simulink model "DC_grid_V2"  (R2018a)
settings: Solver=VariableStepAuto  StartTime=0.0  StopTime=10  RelTol=1e-3
values from neighbouring files (symbols this model uses):
  inputsFromWS = Simulink.Parameter(inputArray)    [DC_grid.m]    (also in QlearningEMS_Average.m; init_for_DC_grid.m)
  Q = repmat(zeros(size(states,1),1,'single'),[1,3,3])    [QlearningEMS.m]    (also in QlearningEMS_Average.m = repmat(zeros(size(Q_states,1),1,'single'),[1,3]))
undefined symbols (not defined in the file or in its folder): Batt, BatteryCback, BatteryLoadFcn, Continuous, FC, FuelCellLoadFcn, gcbh, MC, sps_rtmsupport, spsBatteryModel
libraries: simulink x7, powerlib x6, spsFuelCellModel x1
settings Model: SimulationMode=accelerator  Creator=David Pasdeloup  LastModifiedBy=David Pasdeloup
settings DataIOCC: FinalStateName=myOperPoint  LoadInitialState=on  SaveFinalState=on  SaveCompleteFinalSimState=on

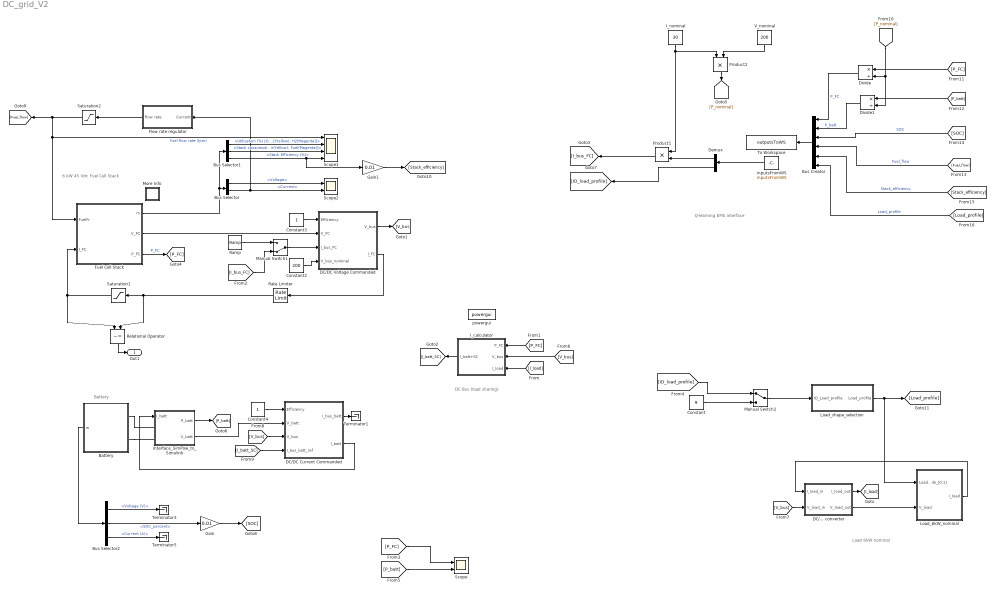
== system DC_grid_V2 ==
  note: 6 kW 45 Vdc Fuel Cell Stack
  note: Battery
  note: DC Bus (load sharing)
  note: Load 6kW nominal
  note: Q-learning EMS interface
  Battery : Subsystem  DialogController=POWERSYS.PowerSysDialog  LoadFcn=sps_rtmsupport('LoadFcn',gcbh); BatteryLoadFcn(gcb)  InitFcn=BatteryCback(gcb,1)  StartFcn=sps_rtmsupport('StartFcn',gcbh);  StopFcn=sps_rtmsupport('StopFcn',gcbh);  mask(Battery){BatType=Lithium-Ion, ShowTempParam=off, ThermalPreset=no, ShowAgeParam=off, NomV=MC.nominal_voltage, NomQ=MC.rated_capacity, SOC=MC.initial_SOC, Batt_Tr=MC.battery_response_time, PresetModel=off, MaxQ=1.5, MinV=75, FullV=116.3987, Dis_rate=64, R=0.66667, Normal_OP=1.3565, expZone=[108.0386    0.07369565], current=100, Units=Time, Tci=20, NomT=25, T2=0, MaxQ2=2.208, FullV2=3.45, Normal_OP2=2.8, expZone2=[3.22        0.23], Rca=0.6, ti=1000, Dp=0, Neq0=0, Tsim=1e6, Ta1=25, Qeol=5.4*0.9, Reol=0.013333*1.2, Char_age=[2.3478, 3], Dis_age=[2.3478, 10], N1=1500, N2=10500, N3=1000, N4=1400, Ta2=45, N5=950}
      mask prompts: BatType "Type:"; ShowTempParam "Simulate temperature effects"; ThermalPreset "Use a preset battery:"; ShowAgeParam "Simulate aging effects"; NomV "Nominal voltage (V)"; NomQ "Rated capacity (Ah)"; SOC "Initial state-of-charge (%)"; Batt_Tr "Battery response time (s)"; PresetModel "Determined from the nominal parameters of the battery"; MaxQ "Maximum capacity (Ah)"; MinV "Cut-off Voltage (V)"; FullV "Fully charged voltage (V)"; Dis_rate "Nominal discharge current (A)"; R "Internal resistance (Ohms)"; Normal_OP "Capacity (Ah) at nominal voltage"; expZone "Exponential zone [Voltage (V), Capacity (Ah)]"; current "Discharge current [i1, i2, i3,...] (A)"; Tci "Initial cell temperature (deg. C)"; NomT "Nominal ambient temperature T1 (deg. C)"; T2 "Second ambient temperature T2 (deg. C)"; MaxQ2 "Maximum capacity (Ah)"; FullV2 "Initial discharge voltage (V)"; Normal_OP2 "Voltage at 90% maximum capacity (V)"; expZone2 "Exponential zone [Voltage (V), Capacity (Ah)]"; Rca "Thermal resistance, cell-to-ambient (deg. C/W)"; ti "Thermal time constant, cell-to-ambient (s)"; Dp "Heat loss difference [charge vs. discharge] (W)"; Neq0 "Initial battery age (Equivalent full cycles)"; Tsim "Aging model sampling time (s)"; Ta1 "Ambient temperature Ta1 (deg. C)"; Qeol "Capacity at EOL (End Of Life) (Ah)"; Reol "Internal resistance at EOL (Ohms)"; Char_age "Charge current (nominal, maximum) [Ic (A), Icmax (A)]"; Dis_age "Discharge current (nominal, maximum) [Id (A), Idmax (A)]"; N1 "Cycle life at 100 % DOD, Ic and Id (Cycles)"; N2 "Cycle life at 25 % DOD, Ic and Id (Cycles)"; N3 "Cycle life at 100 % DOD, Ic and Idmax (Cycles)"; N4 "Cycle life at 100 % DOD, Icmax and Id (Cycles)"; Ta2 "Ambient temperature Ta2 (deg. C)"; N5 "Cycle life at 100 % DOD, Ic and Id (Cycles)"
      mask help: Implements a generic battery model for most popular battery types. Temperature and aging (due to cycling) effects can be specified for Lithium-Ion battery type.
      mask init:
      | block = gcb;
      | BatteryCback(block,3)
      | [Batt BT, WantBlockChoice, Ts] = BatteryParam(NomV,NomQ,MaxQ,MinV,FullV,Dis_rate,R,Normal_OP,expZone,block,0);
      | powericon('SetInternalModels','set',block,WantBlockChoice);
      | BatteryCback(block,1);
      | 
      | % Lines added by David Pasdeloup 27 June 2018
      | %disp('The battery model have been initialized now'); %flag to (un)comment
      settings: CopyFcn=sps_rtmsupport('CopyFcn',gcbh);  DeleteFcn=sps_rtmsupport('DeleteFcn',gcbh);  UndoDeleteFcn=sps_rtmsupport('UndoDeleteFcn',gcbh);  ModelCloseFcn=sps_rtmsupport('ModelCloseFcn',gcbh);  PreSaveFcn=sps_rtmsupport('PreSaveFcn',gcbh);  PostSaveFcn=sps_rtmsupport('PostSaveFcn',gcbh);  NameChangeFcn=sps_rtmsupport('NameChangeFcn',gcbh);  PreCopyFcn=sps_rtmsupport('PreCopyFcn',gcbh);  OpenFcn=sps_rtmsupport('OpenFcn',gcbh, [1,2,3,4,9,18]);  CloseFcn=sps_rtmsupport('CloseFcn',gcbh);  PreDeleteFcn=sps_rtmsupport('PreDeleteFcn',gcbh);
      mask Help: helpview(psbhelp)
      mask TypeOptions BatType: Lead-Acid | Lithium-Ion | Nickel-Cadmium | Nickel-Metal-Hydride
      mask Callback BatType: BatteryCback(gcb,1)
      mask Callback ShowTempParam: BatteryCback(gcb,1)
      mask TypeOptions ThermalPreset: no | 3.3V  2.3Ah  (LiFePO4) | 3.6V  2050mAh   (LiCoO2) | 3.6V  2.0Ah | 3.6V  3.6Ah  (LiNiO2) | 3.6V  4.5Ah | 3.6V  48Ah  (LiNiO2) | 3.7V  4.4Ah | 7.4V  5.4Ah  (LiCoO2) | 11.1V  6600mAh  (LiCoO2) | 12.8V  40Ah  (LiFeMgPO4)
      mask Callback ThermalPreset: BatteryCback(gcb,4)
      mask Callback ShowAgeParam: BatteryCback(gcb,1)
      mask Callback PresetModel: BatteryCback(gcb,1)
      mask TypeOptions Units: Ampere-hour | Time
      mask Callback ti: sps_rtmsupport('parametereditingmodes',gcbh, [1,2,3,4,9,18]);
      mask DialogControl ParameterTabVar0 Prompt: Parameters
      mask DialogControl Tempcontainer Prompt: Temperature
      mask DialogControl Agecontainer Prompt: Aging
      mask DialogControl ParameterTabVar01 Prompt: Discharge
      mask DialogControl Container9 Prompt: Display characteristics
      mask DialogControl PlotButton Prompt: Plot
      mask DialogControl PlotButton Callback: BatteryCback(gcb,0)
      mask DialogControl Temperature Prompt: Temperature
      mask DialogControl Container7 Prompt: Discharge parameters at T2
      mask DialogControl Container8 Prompt: Thermal response and Heat loss
      mask DialogControl Aging Prompt: Aging
      mask DialogControl Container16 Prompt: Aging characteristics at ambient temperature Ta1
      mask DialogControl Container13 Prompt: Aging characteristics at ambient temperature Ta2
      mask Display:
      | patch([BT.X1 BT.X1m],[BT.Y1 BT.Y1m],BT.color1);
      | patch(BT.X3,BT.Y3,BT.color2);
      | plot([BT.X1 BT.X1m BT.X2 BT.X2m BT.X3 BT.X4],[BT.Y1 BT.Y1m BT.Y2 BT.Y2m BT.Y3 BT.Y4]);
      | plot(-100,-60,60,50,[BT.X(1) BT.X(1)],[BT.bas BT.haut],[BT.X(2) BT.X(2)],[BT.haut BT.bas],BT.dim_Xsin,4*sin(BT.dim_sin)+BT.haut,BT.dim_Xsin,-4*sin(BT.dim_sin)+BT.haut,BT.dim_Xsin,-4*sin(BT.dim_sin)+BT.bas,BT.dim_Xtop,sin(BT.dim_top)+BT.haut+4,BT.dim_Xtop,-sin(BT.dim_top)+BT.haut+4,BT.dim_Xtop,-sin(BT.dim_top)+BT.haut,[BT.TopX(2),BT.TopX(2)],[BT.haut,BT.haut+4],[BT.TopX(1),BT.TopX(1)],[BT.haut+4,BT.haut]);plot(BT.dim_Xsin,-5*sin(BT.dim_sin)+20);
      | port_label('lconn',1,'+');
      | port_label('lconn',2,'_');
      | color('blue');
      | port_label('output',1,'m');
      | 
      | if Batt.sel_T
      |     port_label('input',1,'Ta');
      | end
  Bus Creator : BusCreator  Inputs=6
  Bus Selector : BusSelector  OutputSignals=Voltage,Current
  Bus Selector1 : BusSelector  OutputSignals=Utilization (%) [O2(Yellow); H2(Magenta)],Stack consumption (lpm) [Air(Yellow); Fuel(Magenta)],Stack Efficiency (%)
  Bus Selector2 : BusSelector  OutputSignals=Voltage (V),SOC_percent,Current (A)
  Constant : Constant  Value=9
  Constant2 : Constant  Value=200
  Constant3 : Constant
  Constant4 : Constant
  DC/... converter : Subsystem
  DC/DC Current Commanded : Subsystem
  DC/DC Voltage Commanded : Subsystem
  Demux : Demux  Outputs=2
  Divide : Product  Inputs=*/
  Divide1 : Product  Inputs=*/
  Flow rate regulator : Subsystem  mask{Nc=65, Uf_H2=99.56, T=65, Pf=1.5, x=99.95}
      mask prompts: Nc "Number of cells"; Uf_H2 "Nominal Hydrogen utilization (%)"; T "Operating temperature (Celsius)"; Pf "Fuel pressure (bar)"; x "H2 composition (%)"
  Fuel Cell Stack : Subsystem  DialogController=POWERSYS.PowerSysDialog  LoadFcn=sps_rtmsupport('LoadFcn',gcbh);FuelCellLoadFcn(gcb)  StartFcn=sps_rtmsupport('StartFcn',gcbh);  StopFcn=sps_rtmsupport('StopFcn',gcbh);  mask(Fuel Cell Stack){PresetModel=PEMFC - 6 kW - 45 Vdc, FcType=Proton Exchange Membrane (PEM), Detailed=Detailed, Eoc=[65,63], NomVI=[133.3,45], EndVI=[225,37], Nc=65, n=55, TOp=65, AirFr=300, SuppPress=[1.5,1], Comp=[99.95,21,1], SignX=off, SignY=off, FlowRateH2=on, FlowRateAir=off, SystemTemp=off, SystemPH2=off, SystemPAir=off, FCDyn=on, FC_tau=10, Peak_O2=80, V_Under=10}
      mask prompts: PresetModel "Preset model:"; FcType "Fuel Cell type:"; Detailed "Model detail Level:"; Eoc "Voltage at 0A and 1A [V_0(V), V_1(V)]"; NomVI "Nominal operating point [Inom(A), Vnom(V)]"; EndVI "Maximum operating point [Iend(A), Vend(V)]"; Nc "Number of cells"; n "Nominal stack efficiency (%)"; TOp "Operating temperature (Celsius)"; AirFr "Nominal Air flow rate (lpm)"; SuppPress "Nominal supply pressure [Fuel (bar), Air (bar)]"; Comp "Nominal composition (%) [H2 O2 H2O(Air)]"; SignX "Fuel  composition [x_H2(%)]"; SignY "Oxidant composition [y_O2(%)]"; FlowRateH2 "Fuel flow rate [FuelFr(lpm)]"; FlowRateAir "Air flow rate [AirFr(lpm)]"; SystemTemp "System Temperature [T(Kelvin)]"; SystemPH2 "Fuel supply pressure [Pfuel(bar)]"; SystemPAir "Air supply pressure [PAir(bar)]"; FCDyn "Specify Fuel Cell Dynamics?"; FC_tau "Fuel Cell response time (sec)"; Peak_O2 "Peak O2 utilization (%)"; V_Under "Voltage undershoot (V) @ peak O2 utilization"
      mask help:
      | Implements a generic hydrogen fuel cell model which allows the simulation for the following types of cells:
      | - Proton Exchange Membrane Fuel Cell (PEMFC)
      | - Solid Oxide Fuel Cell (SOFC)
      | - Alkaline Fuel Cell (AFC)
      mask init:
      | block = gcb;
      | %% DO NOT CHANGE THIS ORDER
      | FuelCellCback(block,'Inputs')
      | [FC, WantBlockChoice, Ts] = FuelCellInit(block,Eoc,NomVI,EndVI,Nc,n,TOp,AirFr,SuppPress,Comp,FlowRateH2,FlowRateAir);
      | powericon('SetInternalModels','set',block,WantBlockChoice);
      | 
      | % Added by David 27/06/2018. Uncomment this line to track when the 
      | % model is compilled:
      | %disp('FC has been initilaized');
      settings: CopyFcn=sps_rtmsupport('CopyFcn',gcbh);  DeleteFcn=sps_rtmsupport('DeleteFcn',gcbh);  UndoDeleteFcn=sps_rtmsupport('UndoDeleteFcn',gcbh);  ModelCloseFcn=sps_rtmsupport('ModelCloseFcn',gcbh);  PreSaveFcn=sps_rtmsupport('PreSaveFcn',gcbh);  PostSaveFcn=sps_rtmsupport('PostSaveFcn',gcbh);  NameChangeFcn=sps_rtmsupport('NameChangeFcn',gcbh);  PreCopyFcn=sps_rtmsupport('PreCopyFcn',gcbh);  OpenFcn=sps_rtmsupport('OpenFcn',gcbh, [1 2 3 13 14 15 16 17 18 19 20]);  CloseFcn=sps_rtmsupport('CloseFcn',gcbh);  PreDeleteFcn=sps_rtmsupport('PreDeleteFcn',gcbh);
      mask Help: helpview(psbhelp)
      mask TypeOptions PresetModel: No (User-Defined) | PEMFC - 1.26 kW - 24 Vdc | PEMFC - 6 kW - 45 Vdc | PEMFC - 50 kW - 625 Vdc | AFC - 2.4 kW - 48 Vdc | SOFC - 3 kW - 100 Vdc | SOFC - 25 kW - 630 Vdc
      mask Callback PresetModel: FuelCellCback(gcb,'Preset')
      mask TypeOptions Detailed: Simplified | Detailed
      mask Callback Detailed: FuelCellCback(gcb,'Visibilities')
      mask Callback FlowRateAir: FuelCellCback(gcb,'Visibilities')
      mask Callback FCDyn: FuelCellCback(gcb,'Visibilities')
      mask DialogControl ParameterTabVar0 Prompt: Parameters
      mask DialogControl plot_graph Prompt: Plot V_I characteristic
      mask DialogControl plot_graph Callback: FuelCellCback(gcb,'PlotGraph');
      mask DialogControl ViewParam Prompt: View Cell parameters
      mask DialogControl ViewParam Callback: FuelCellCback(gcb,'ViewParam');
      mask DialogControl ParameterTabVar01 Prompt: Signal variation
      mask DialogControl ParameterTabVar012 Prompt: Fuel Cell Dynamics
      mask Display: image(imread('power_fuelcell.png'));
  Gain : Gain  Gain=0.01
  Gain1 : Gain  Gain=0.01
  I_calculator : Subsystem
  I_nominal : Constant  Value=30
  Interface_SimPow_to_Simulink : Subsystem
  Load_6kW_nominal : Subsystem
  Load_shape_selection : Subsystem
  Manual Switch1 : ManualSwitch  CurrentSetting=0
  Manual Switch2 : ManualSwitch
  More Info : Subsystem
      settings: OpenFcn=showdemo(bdroot(gcb))
      mask Display: disp('?')
  Product1 : Product
  Product2 : Product
  Ramp : simulink/Sources/Ramp  slope=5  start=10  InitialOutput=0
  Rate Limiter : RateLimiter  RisingSlewLimit=8  FallingSlewLimit=-8  SampleTimeMode=inherited
  Relational Operator : RelationalOperator  Operator=~=  OutDataTypeStr=boolean  RndMeth=Simplest
  Saturation1 : Saturate  UpperLimit=225  LowerLimit=0
  Saturation2 : Saturate  UpperLimit=85  LowerLimit=0
  Scope : Scope  NumInputPorts=2
  Scope1 : Scope  NumInputPorts=4
  Scope2 : Scope  NumInputPorts=2
  Terminator1 : Terminator
  Terminator3 : Terminator
  Terminator5 : Terminator
  To Workspace : ToWorkspace  VariableName=outputsToWS  SaveFormat=Timeseries  SampleTime=-1
  V_nominal : Constant  Value=200
  inputsFromWS : Constant  Value=inputsFromWS
  powergui : powerlib/powergui  SimulationMode=Continuous  SampleTime=1e-6  frequency=60  Iterations=50  frequencyindice=0  Pbase=100e6  ErrMax=1e-4  UnitsV=kV  UnitsW=MW  buscounter=0  FunctionMessages=off  echomessages=off  EnableUseOfTLC=off  CurrentSourceSwitches=off  DisableSnubberDevices=off  DisableRonSwitches=off  DisableVfSwitches=off  DisplayEquations=off  SolverType=Tustin/Backward Euler (TBE)  Interpol=off  ExternalGateDelay=off  methode=off  Ts=100  x0status=blocks  SPID=on  SwTol=0  HookPort=off  RestoreLinks=warning  ResistiveCurrentMeasurement=off  Frange=[0:2:500]  Ylog=off  Xlog=on  ShowGrid=off  save=off  variable=ZData  structure=0  ZoomFFT=on  StartTime=0.0  cycles=1  DisplayStyle=1  fundamental=60  FreqAxis=off  MaxFrequency=1000  frequencyindicesteady=1  RmsSteady=1  display=off
  Out1 : Outport
  wires:
  Battery/1(m) -> Bus Selector2/1
  Constant2/1 -> DC/DC Voltage Commanded/4(V_bus_nominal)
  [I_bus_FC] -> Manual Switch1/2
  Constant/1 -> Manual Switch2/2
  Manual Switch1/1 -> DC/DC Voltage Commanded/3(I_bus_FC)
  [ID_load_profile] -> Manual Switch2/1
  Interface_SimPow_to_Simulink/1(P_batt) -> [P_batt]
  Fuel Cell Stack/1(m) -> Bus Selector/1, Bus Selector1/1
  Load_6kW_nominal/1(I_load) -> DC/... converter/1(I_load_in)
  Saturation1/1 -> Relational Operator/1, Fuel Cell Stack/2(I_FC)
  [I_load] -> I_calculator/3(I_load)
  Relational Operator/1 -> Out1/1
  DC/... converter/1(I_load_out) -> [I_load]
  Rate Limiter/1 -> Relational Operator/2, Saturation1/1
  Constant3/1 -> DC/DC Voltage Commanded/1(Efficiency)
  Bus Selector1/1 -> Scope1/2  "<Utilization (%) [O2(Yellow); H2(Magenta)]>"
  Ramp/1 -> Manual Switch1/1
  DC/DC Voltage Commanded/2(I_FC) -> Rate Limiter/1
  Bus Selector1/2 -> Scope1/3  "<Stack consumption (lpm) [Air(Yellow); Fuel(Magenta)]>"
  DC/... converter/2(V_load_out) -> Load_6kW_nominal/2(V_load)
  Fuel Cell Stack/3(P_FC) -> [P_FC]  "P_FC"
  Saturation2/1 -> [Fuel_flow], Fuel Cell Stack/1(FuelFr), Scope1/1  "Fuel flow rate (lpm)"
  Bus Selector1/3 -> Gain1/1, Scope1/4  "<Stack Efficiency (%)>"
  Bus Selector/2 -> Flow rate regulator/1(Current), Scope2/2  "<Current>"
  Bus Selector/1 -> Scope2/1  "<Voltage>"
  Flow rate regulator/1(flow rate) -> Saturation2/1
  Bus Selector2/3 -> Terminator5/1  "<Current (A)>"
  Bus Selector2/2 -> Gain/1  "<SOC_percent>"
  Bus Selector2/1 -> Terminator3/1  "<Voltage (V)>"
  [P_FC] -> Scope/1
  [P_batt] -> Scope/2
  Constant4/1 -> DC/DC Current Commanded/1(Efficiency)
  Interface_SimPow_to_Simulink/2(V_batt) -> DC/DC Current Commanded/2(V_batt)
  DC/DC Current Commanded/2(I_batt) -> Interface_SimPow_to_Simulink/1(I_batt)
  DC/DC Current Commanded/1(I_bus_batt) -> Terminator1/1
  [P_FC] -> I_calculator/1(P_FC)
  DC/DC Voltage Commanded/1(V_bus) -> [V_bus]
  [V_bus] -> I_calculator/2(V_bus)
  Fuel Cell Stack/2(V_FC) -> DC/DC Voltage Commanded/2(V_FC)
  [V_bus] -> DC/... converter/2(V_load_in)
  [V_bus] -> DC/DC Current Commanded/3(V_bus)
  I_calculator/1(I_batt+SC) -> [I_batt_SC]
  [I_batt_SC] -> DC/DC Current Commanded/4(I_bus_batt_ref)
  Demux/1 -> Product1/2
  Demux/2 -> [ID_load_profile]
  Bus Creator/1 -> To Workspace/1
  [P_batt] -> Divide1/1
  Divide1/1 -> Bus Creator/2  "P_batt"
  inputsFromWS/1 -> Demux/1
  Product1/1 -> [I_bus_FC]
  Divide/1 -> Bus Creator/1  "P_FC"
  Product2/1 -> [P_nominal]
  [P_nominal] -> Divide1/2, Divide/2
  V_nominal/1 -> Product2/2
  [P_FC] -> Divide/1
  I_nominal/1 -> Product1/1, Product2/1
  [SOC] -> Bus Creator/3  "SOC"
  Gain/1 -> [SOC]
  Gain1/1 -> [Stack_efficiency]
  [Fuel_flow] -> Bus Creator/4  "Fuel_flow"
  [Stack_efficiency] -> Bus Creator/5  "Stack_efficiency"
  Manual Switch2/1 -> Load_shape_selection/1(ID_Load_profile)
  Load_shape_selection/1(Load_profile) -> [Load_profile], Load_6kW_nominal/1(Load_profile_[0;1])
  [Load_profile] -> Bus Creator/6  "Load_profile"
  connections:
  Battery/LConn2 -- Interface_SimPow_to_Simulink/LConn2
  Battery/LConn1 -- Interface_SimPow_to_Simulink/LConn1

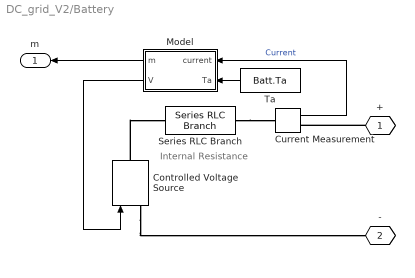
== system DC_grid_V2/Battery ==
  note: Internal Resistance
  Controlled Voltage Source : powerlib/Electrical Sources/Controlled Voltage Source  Initialize=on  Source_Type=AC  Amplitude=0  Phase=0  Frequency=0  Measurements=None
  Current Measurement : powerlib/Measurements/Current Measurement  PhasorSimulation=off  OutputType=Complex  PSBequivalent=0
  Model : Subsystem  AncestorBlock=spsBatteryModel/Continuous
  Series RLC Branch : powerlib/Elements/Series RLC Branch  LConnTagsString=__new0  RConnTagsString=__new0  BranchType=R  Resistance=Batt.R  Inductance=1e-3  SetiL0=off  InitialCurrent=0  Capacitance=1e-6  Setx0=off  InitialVoltage=0  Measurements=None
  Ta : Constant  Value=Batt.Ta
  + : PMIOPort  Tag=PMCPort  Side=Left
  - : PMIOPort  Tag=PMCPort  Port=2  Side=Left
  m : Outport
  wires:
  Ta/1 -> Model/2(Ta)
  Current Measurement/1 -> Model/1(current)  "Current"
  Model/1(m) -> m/1
  Model/2(V) -> Controlled Voltage Source/1
  connections:
  Series RLC Branch/RConn1 -- Current Measurement/LConn1
  Controlled Voltage Source/RConn1 -- Series RLC Branch/LConn1
  Controlled Voltage Source/LConn1 -- -/RConn1
  +/RConn1 -- Current Measurement/RConn1

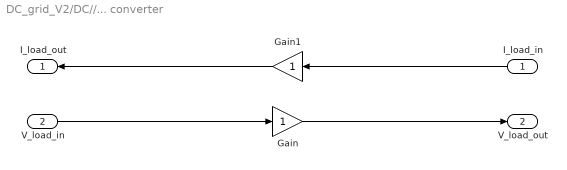
== system DC_grid_V2/DC//... converter ==
  I_load_in : Inport
  V_load_in : Inport  Port=2
  Gain : Gain
  Gain1 : Gain
  I_load_out : Outport
  V_load_out : Outport  Port=2
  wires:
  I_load_in/1 -> Gain1/1
  Gain/1 -> V_load_out/1
  Gain1/1 -> I_load_out/1
  V_load_in/1 -> Gain/1

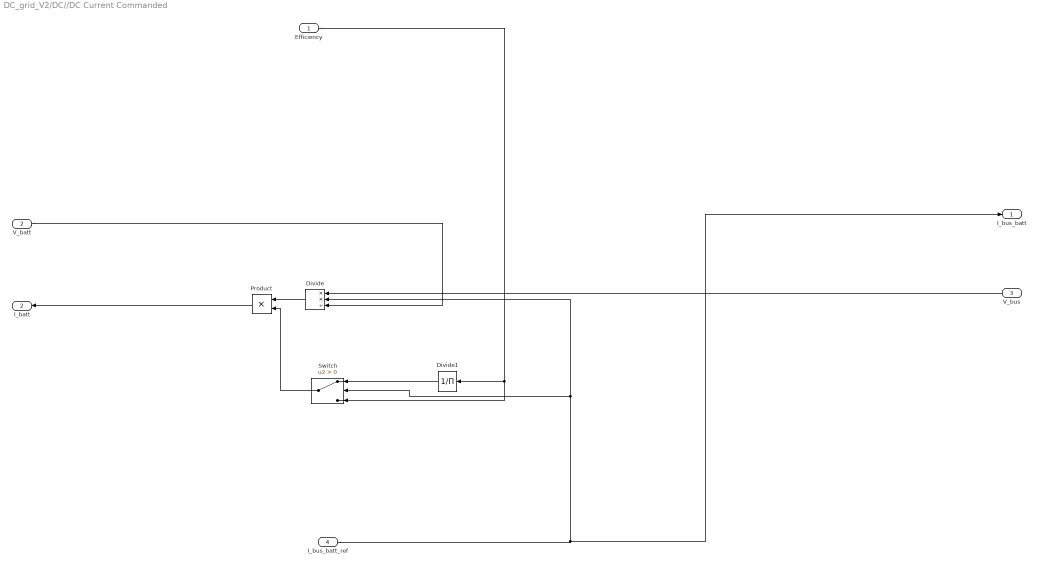
== system DC_grid_V2/DC//DC Current Commanded ==
  Efficiency : Inport
  V_batt : Inport  Port=2
  V_bus : Inport  Port=3
  I_bus_batt_ref : Inport  Port=4
  Divide : Product  Inputs=**/
  Divide1 : Product  Inputs=/
  Product : Product
  Switch : Switch  Criteria=u2 > Threshold
  I_bus_batt : Outport
  I_batt : Outport  Port=2
  wires:
  I_bus_batt_ref/1 -> Divide/2, Switch/2, I_bus_batt/1
  V_bus/1 -> Divide/1
  V_batt/1 -> Divide/3
  Efficiency/1 -> Divide1/1, Switch/3
  Divide1/1 -> Switch/1
  Divide/1 -> Product/1
  Switch/1 -> Product/2
  Product/1 -> I_batt/1

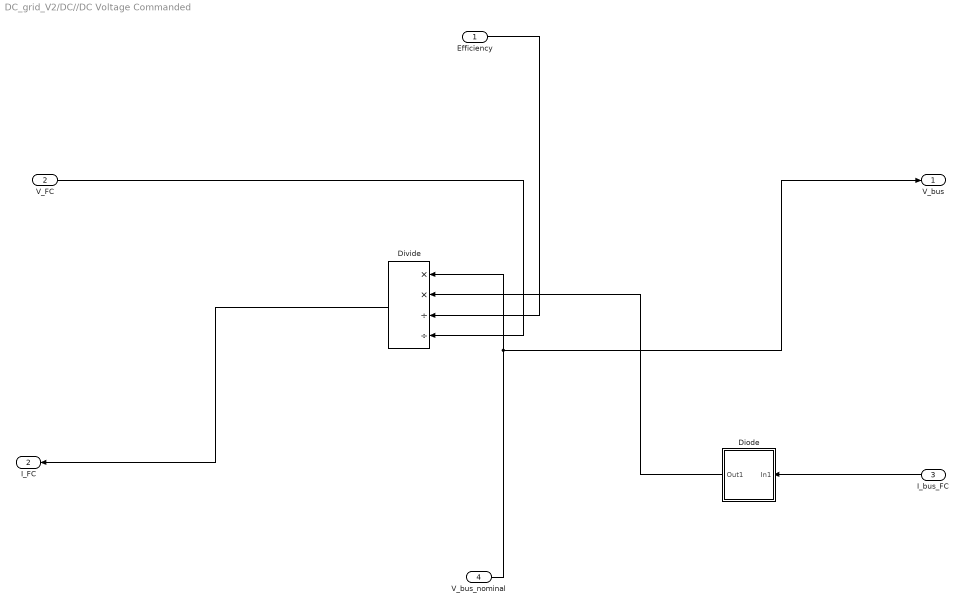
== system DC_grid_V2/DC//DC Voltage Commanded ==
  Efficiency : Inport
  V_FC : Inport  Port=2
  I_bus_FC : Inport  Port=3
  V_bus_nominal : Inport  Port=4
  Diode : Subsystem
  Divide : Product  Inputs=**//
  V_bus : Outport
  I_FC : Outport  Port=2
  wires:
  V_bus_nominal/1 -> V_bus/1, Divide/1
  V_FC/1 -> Divide/4
  Divide/1 -> I_FC/1
  Efficiency/1 -> Divide/3
  I_bus_FC/1 -> Diode/1(In1)
  Diode/1(Out1) -> Divide/2

== system DC_grid_V2/Flow rate regulator ==
  Current : Inport
  Fcn1 : Fcn  Expr=60000*8.3145*(273+T)*Nc*u(1)/(2*96485*(Pf*101325)*Uf_H2/100*x/100)
  Saturation : Saturate  UpperLimit=inf  LowerLimit=1
  flow rate : Outport
  wires:
  Fcn1/1 -> Saturation/1
  Current/1 -> Fcn1/1
  Saturation/1 -> flow rate/1

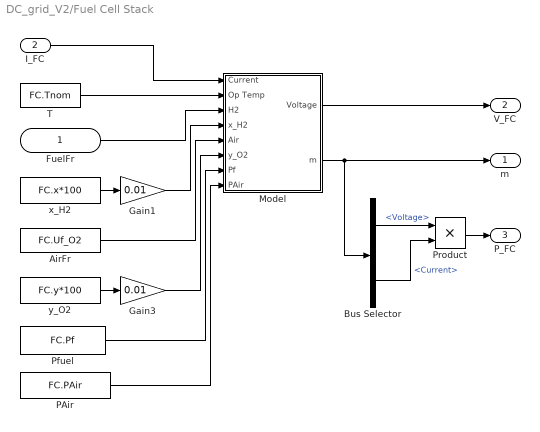
== system DC_grid_V2/Fuel Cell Stack ==
  FuelFr : Inport
  I_FC : Inport  Port=2
  AirFr : Constant  Value=FC.Uf_O2
  Bus Selector : BusSelector  OutputSignals=Voltage,Current
  Gain1 : Gain  Gain=0.01
  Gain3 : Gain  Gain=0.01
  Model : Subsystem  BlockChoice=Continuous/Detailed
      settings: AttributesFormatString=%<BlockChoice>  TemplateBlock=spsFuelCellModel/Fuel Cell model  MemberBlocks=Continuous/Detailed,Continuous/Simplified,Discrete/Detailed,Discrete/Simplified
  PAir : Constant  Value=FC.PAir
  Pfuel : Constant  Value=FC.Pf
  Product : Product
  T : Constant  Value=FC.Tnom
  x_H2 : Constant  Value=FC.x*100
  y_O2 : Constant  Value=FC.y*100
  m : Outport
  V_FC : Outport  Port=2
  P_FC : Outport  Port=3
  wires:
  PAir/1 -> Model/8(PAir)
  Pfuel/1 -> Model/7(Pf)
  T/1 -> Model/2(Op Temp)
  Model/1(Voltage) -> V_FC/1
  Model/2(m) -> Bus Selector/1, m/1
  FuelFr/1 -> Model/3(H2)
  x_H2/1 -> Gain1/1
  AirFr/1 -> Model/5(Air)
  y_O2/1 -> Gain3/1
  Gain1/1 -> Model/4(x_H2)
  Gain3/1 -> Model/6(y_O2)
  I_FC/1 -> Model/1(Current)
  Bus Selector/1 -> Product/1  "<Voltage>"
  Bus Selector/2 -> Product/2  "<Current>"
  Product/1 -> P_FC/1

== system DC_grid_V2/I_calculator ==
  P_FC : Inport
  V_bus : Inport  Port=2
  I_load : Inport  Port=3
  Add : Sum  Inputs=-+
  Divide : Product  Inputs=*/
  I_batt+SC : Outport
  wires:
  I_load/1 -> Add/2
  Divide/1 -> Add/1
  P_FC/1 -> Divide/1
  V_bus/1 -> Divide/2
  Add/1 -> I_batt+SC/1

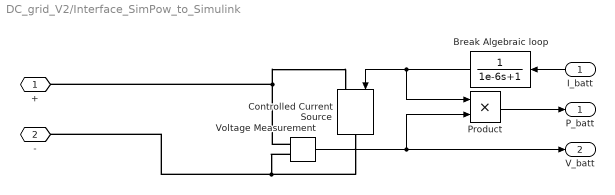
== system DC_grid_V2/Interface_SimPow_to_Simulink ==
  I_batt : Inport
  Break Algebraic loop : TransferFcn  Denominator=[1e-6 1]
  Controlled Current Source : powerlib/Electrical Sources/Controlled Current Source  Initialize=off  Source_Type=DC  Amplitude=0  Phase=0  Frequency=0  Measurements=None
  Product : Product
  Voltage Measurement : powerlib/Measurements/Voltage Measurement  PhasorSimulation=off  OutputType=Complex  PSBequivalent=0
  + : PMIOPort  Side=Left
  - : PMIOPort  Port=2  Side=Left
  P_batt : Outport
  V_batt : Outport  Port=2
  wires:
  Product/1 -> P_batt/1
  I_batt/1 -> Break Algebraic loop/1
  Voltage Measurement/1 -> V_batt/1, Product/2
  Break Algebraic loop/1 -> Product/1, Controlled Current Source/1
  connections:
  Voltage Measurement/LConn2 -- Controlled Current Source/RConn1 -- -/RConn1
  Voltage Measurement/LConn1 -- Controlled Current Source/LConn1 -- +/RConn1

== system DC_grid_V2/Load_6kW_nominal ==
  Load_profile_[0;1] : Inport
  V_load : Inport  Port=2
  I=P/U : Product  Inputs=*/
  Nominal_load_power : Constant  Value=6000
  Product : Product
  I_load : Outport
  wires:
  Load_profile_[0;1]/1 -> Product/2
  Product/1 -> I=P/U/1
  Nominal_load_power/1 -> Product/1
  V_load/1 -> I=P/U/2
  I=P/U/1 -> I_load/1

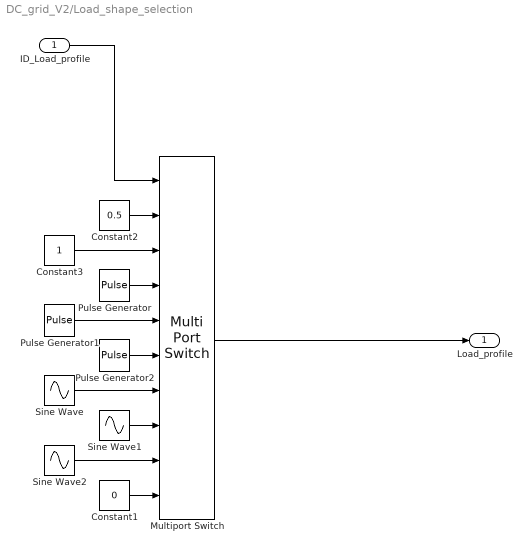
== system DC_grid_V2/Load_shape_selection ==
  ID_Load_profile : Inport
  Constant1 : Constant  Value=0
  Constant2 : Constant  Value=0.5
  Constant3 : Constant
  Multiport Switch : MultiPortSwitch  DataPortOrder=Specify indices  DataPortIndices={1,2,3,4,5,6,7,8,9}
  Pulse Generator : DiscretePulseGenerator  PulseType=Time based  Period=1  PulseWidth=50  PhaseDelay=10
  Pulse Generator1 : DiscretePulseGenerator  PulseType=Time based  Period=5  PulseWidth=50  PhaseDelay=10
  Pulse Generator2 : DiscretePulseGenerator  PulseType=Time based  Period=60  PulseWidth=50  PhaseDelay=10
  Sine Wave : Sin  Amplitude=0.5  Bias=0.5  Frequency=2*pi  Phase=-pi/2  SampleTime=0
  Sine Wave1 : Sin  Amplitude=0.5  Bias=0.5  Frequency=2*pi/5  Phase=-pi/2  SampleTime=0
  Sine Wave2 : Sin  Amplitude=0.5  Bias=0.5  Frequency=2*pi/60  Phase=-pi/2  SampleTime=0
  Load_profile : Outport
  wires:
  Constant1/1 -> Multiport Switch/10
  Sine Wave2/1 -> Multiport Switch/9
  Pulse Generator2/1 -> Multiport Switch/6
  Sine Wave/1 -> Multiport Switch/7
  Constant2/1 -> Multiport Switch/2
  Constant3/1 -> Multiport Switch/3
  Pulse Generator1/1 -> Multiport Switch/5
  Pulse Generator/1 -> Multiport Switch/4
  Sine Wave1/1 -> Multiport Switch/8
  Multiport Switch/1 -> Load_profile/1
  ID_Load_profile/1 -> Multiport Switch/1

== system DC_grid_V2/More Info ==

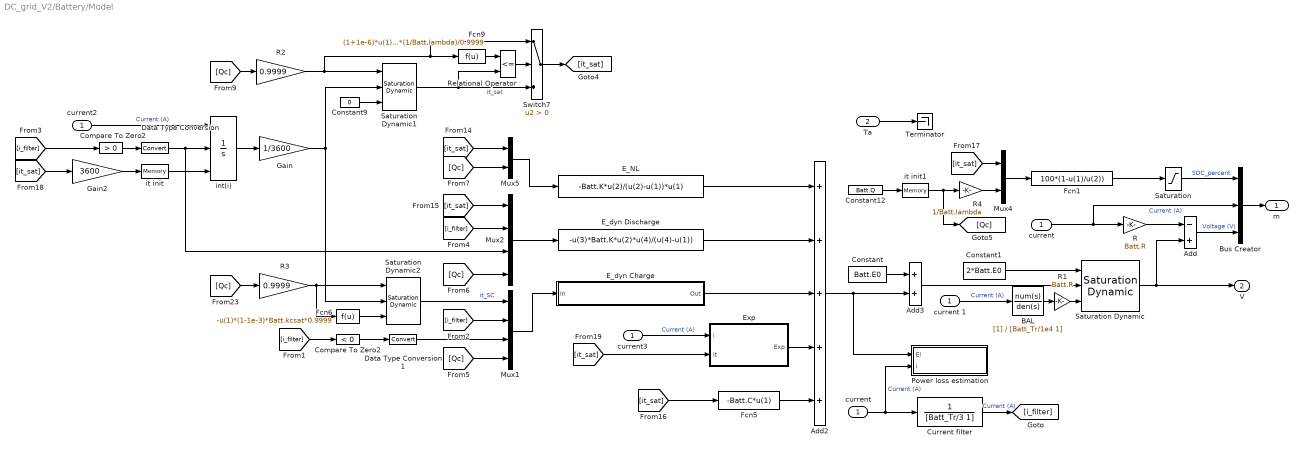
== system DC_grid_V2/Battery/Model ==
  current : Inport
  Ta : Inport  Port=2
  Add : Sum  Inputs=-+
  Add2 : Sum  Inputs=+++++
  Add3 : Sum
  BAL : TransferFcn  Denominator=[Batt_Tr/1e4 1]
  Bus Creator : BusCreator  Inputs=3
  Compare To Zero : simulink/Logic and Bit Operations/Compare To Zero  relop=>  OutDataTypeStr=uint8
  Compare To Zero2 : simulink/Logic and Bit Operations/Compare To Zero  relop=<  OutDataTypeStr=uint8
  Constant : Constant  Value=Batt.E0
  Constant1 : Constant  Value=2*Batt.E0
  Constant12 : Constant  Value=Batt.Q
  Constant9 : Constant  Value=0
  Current filter : TransferFcn  Denominator=[Batt_Tr/3 1]
  Data Type Conversion1 : DataTypeConversion
  Data Type Conversion2 : DataTypeConversion
  E_NL : Fcn  Expr=-Batt.K*u(2)/(u(2)-u(1))*u(1)
  E_dyn Charge : Subsystem
  E_dyn Discharge : Fcn  Expr=-u(3)*Batt.K*u(2)*u(4)/(u(4)-u(1))
  Exp : Subsystem
  Fcn1 : Fcn  Expr=100*(1-u(1)/u(2))
  Fcn5 : Fcn  Expr=-Batt.C*u(1)
  Fcn6 : Fcn  Expr=-u(1)*(1-1e-3)*Batt.kcsat*0.9999
  Fcn9 : Fcn  Expr=(1+1e-6)*u(1)*(1/Batt.lambda)/0.9999
  Gain : Gain  Gain=1/3600
  Gain2 : Gain  Gain=3600
  Mux1 : Mux
  Mux2 : Mux
  Mux4 : Mux  Inputs=2
  Mux5 : Mux  Inputs=2
  Power loss estimation : Subsystem
  R : Gain  Gain=Batt.R
  R1 : Gain  Gain=Batt.R
  R2 : Gain  Gain=0.9999
  R3 : Gain  Gain=0.9999
  R4 : Gain  Gain=1/Batt.lambda
  Relational Operator : RelationalOperator  Operator=<=  RndMeth=Simplest
  Saturation : Saturate  UpperLimit=100  LowerLimit=0
  Saturation Dynamic : simulink/Discontinuities/Saturation Dynamic  OutMin=[]  OutMax=[]  OutDataTypeStr=Inherit: Same as second input  OutDataType=sfix(16)  OutScaling=2^-10  DoSatur=off
  Saturation Dynamic1 : simulink/Discontinuities/Saturation Dynamic  OutMin=[]  OutMax=[]  OutDataTypeStr=Inherit: Same as second input  OutDataType=sfix(16)  OutScaling=2^-10  DoSatur=off
  Saturation Dynamic2 : simulink/Discontinuities/Saturation Dynamic  OutMin=[]  OutMax=[]  OutDataTypeStr=Inherit: Same as second input  OutDataType=sfix(16)  OutScaling=2^-10  DoSatur=off
  Switch7 : Switch  Criteria=u2 > Threshold
  Terminator : Terminator
  "current " : InportShadow
  current 1 : InportShadow
  current2 : InportShadow
  current3 : InportShadow
  int(i) : Integrator  ExternalReset=rising  InitialConditionSource=external  InitialCondition=(1-SOC/100)*Q*3600  LimitOutput=on  UpperSaturationLimit=Batt.Qmax*3600
  it init : Memory  InitialCondition=(1-SOC/100)*Batt.Q*(1/Batt.lambda)*3600
  it init1 : Memory  InitialCondition=Batt.Q
  m : Outport
  V : Outport  Port=2
  wires:
  BAL/1 -> R1/1
  current 1/1 -> BAL/1  "Current (A)"
  Constant12/1 -> it init1/1
  Constant1/1 -> Saturation Dynamic/1
  Ta/1 -> Terminator/1
  current/1 -> R/1, Bus Creator/2  "Current (A)"
  int(i)/1 -> Gain/1
  Fcn1/1 -> Saturation/1
  Add/1 -> Bus Creator/3  "Voltage (V)"
  R/1 -> Add/1
  Bus Creator/1 -> m/1
  Mux2/1 -> E_dyn Discharge/1
  Constant/1 -> Add3/1
  Mux1/1 -> E_dyn Charge/1(In)
  it init/1 -> int(i)/3
  Compare To Zero/1 -> Data Type Conversion2/1
  Compare To Zero2/1 -> Data Type Conversion1/1
  Data Type Conversion2/1 -> Mux2/3, int(i)/2
  Gain2/1 -> it init/1
  Exp/1(Exp) -> Add2/4
  Data Type Conversion1/1 -> Mux1/3
  Saturation Dynamic2/1 -> Mux1/1  "it_SC"
  Add3/1 -> Saturation Dynamic/2
  E_dyn Discharge/1 -> Add2/2
  E_NL/1 -> Add2/1
  E_dyn Charge/1(Out) -> Add2/3
  Fcn5/1 -> Add2/5
  Mux4/1 -> Fcn1/1
  Mux5/1 -> E_NL/1
  Fcn6/1 -> Saturation Dynamic2/3
  current2/1 -> int(i)/1  "Current (A)"
  current3/1 -> Exp/1(i)  "Current (A)"
  "current "/1 -> Current filter/1, Power loss estimation/2(i)  "Current (A)"
  [i_filter] -> Compare To Zero2/1
  [i_filter] -> Mux1/2
  [i_filter] -> Compare To Zero/1
  [i_filter] -> Mux2/2
  [Qc] -> Mux1/4
  [Qc] -> Mux2/4
  it init1/1 -> R4/1, [Qc]
  [Qc] -> R2/1
  [it_sat] -> Mux5/1
  [it_sat] -> Mux2/1
  [it_sat] -> Fcn5/1
  [it_sat] -> Mux4/1
  [it_sat] -> Gain2/1
  [it_sat] -> Exp/2(it)
  [Qc] -> R3/1
  R3/1 -> Fcn6/1, Saturation Dynamic2/1
  Add2/1 -> Add3/2, Power loss estimation/1(El)
  R4/1 -> Mux4/2
  Saturation/1 -> Bus Creator/1  "SOC_percent"
  Saturation Dynamic/1 -> Add/2, V/1
  [Qc] -> Mux5/2
  Gain/1 -> Saturation Dynamic1/2, Saturation Dynamic2/2
  Constant9/1 -> Saturation Dynamic1/3
  Current filter/1 -> [i_filter]  "Current (A)"
  R1/1 -> Saturation Dynamic/3
  Saturation Dynamic1/1 -> Relational Operator/2, Switch7/3  "it_sat"
  R2/1 -> Switch7/1, Fcn9/1, Saturation Dynamic1/1
  Switch7/1 -> [it_sat]
  Fcn9/1 -> Relational Operator/1
  Relational Operator/1 -> Switch7/2

== system DC_grid_V2/DC//DC Voltage Commanded/Diode ==
  In1 : Inport
  Constant : Constant  Value=0
  MinMax : MinMax  Function=max  Inputs=2
  Out1 : Outport
  wires:
  Constant/1 -> MinMax/2
  In1/1 -> MinMax/1
  MinMax/1 -> Out1/1

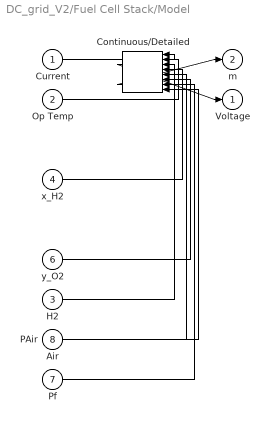
== system DC_grid_V2/Fuel Cell Stack/Model ==
  Current : Inport
  Op Temp : Inport  Port=2
  H2 : Inport  Port=3
  x_H2 : Inport  Port=4
  Air : Inport  Port=5
  y_O2 : Inport  Port=6
  Pf : Inport  Port=7
  PAir : Inport  Port=8
  Continuous/Detailed : spsFuelCellModel/Continuous//Detailed
  Voltage : Outport
  m : Outport  Port=2
  wires:
  Current/1 -> Continuous/Detailed/1
  Op Temp/1 -> Continuous/Detailed/2
  H2/1 -> Continuous/Detailed/3
  x_H2/1 -> Continuous/Detailed/4
  Air/1 -> Continuous/Detailed/5
  y_O2/1 -> Continuous/Detailed/6
  Pf/1 -> Continuous/Detailed/7
  PAir/1 -> Continuous/Detailed/8
  Continuous/Detailed/1 -> Voltage/1
  Continuous/Detailed/2 -> m/1

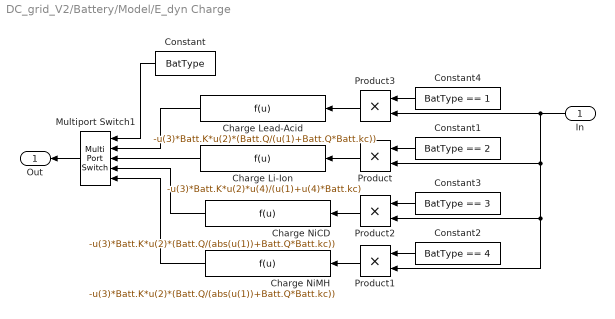
== system DC_grid_V2/Battery/Model/E_dyn Charge ==
  In : Inport
  Charge Lead-Acid : Fcn  Expr=-u(3)*Batt.K*u(2)*(Batt.Q/(u(1)+Batt.Q*Batt.kc))
  Charge Li-Ion : Fcn  Expr=-u(3)*Batt.K*u(2)*u(4)/(u(1)+u(4)*Batt.kc)
  Charge NiCD : Fcn  Expr=-u(3)*Batt.K*u(2)*(Batt.Q/(abs(u(1))+Batt.Q*Batt.kc))
  Charge NiMH : Fcn  Expr=-u(3)*Batt.K*u(2)*(Batt.Q/(abs(u(1))+Batt.Q*Batt.kc))
  Constant : Constant  Value=BatType
  Constant1 : Constant  Value=BatType == 2  OutDataTypeStr=double
  Constant2 : Constant  Value=BatType == 4  OutDataTypeStr=double
  Constant3 : Constant  Value=BatType == 3  OutDataTypeStr=double
  Constant4 : Constant  Value=BatType == 1  OutDataTypeStr=double
  Multiport Switch1 : MultiPortSwitch  Inputs=4
  Product{,1..3} (4 alike) : Product  RndMeth=Zero
  Out : Outport
  wires:
  Multiport Switch1/1 -> Out/1
  Charge Li-Ion/1 -> Multiport Switch1/3
  Charge NiMH/1 -> Multiport Switch1/5
  Charge NiCD/1 -> Multiport Switch1/4
  Charge Lead-Acid/1 -> Multiport Switch1/2
  Constant/1 -> Multiport Switch1/1
  In/1 -> Product3/2, Product/2, Product1/2, Product2/2
  Product/1 -> Charge Li-Ion/1
  Constant1/1 -> Product/1
  Product1/1 -> Charge NiMH/1
  Constant2/1 -> Product1/1
  Product2/1 -> Charge NiCD/1
  Constant3/1 -> Product2/1
  Product3/1 -> Charge Lead-Acid/1
  Constant4/1 -> Product3/1

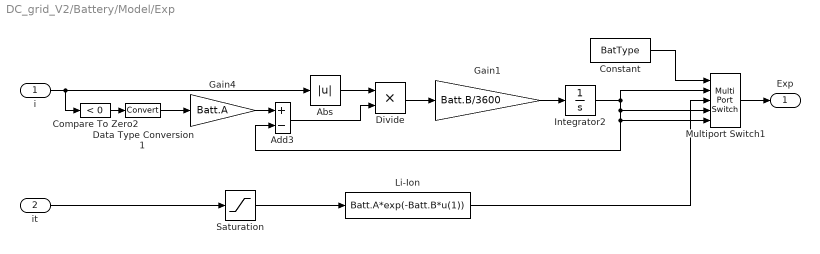
== system DC_grid_V2/Battery/Model/Exp ==
  i : Inport
  it : Inport  Port=2
  Abs : Abs
  Add3 : Sum  Inputs=+-
  Compare To Zero2 : simulink/Logic and Bit Operations/Compare To Zero  relop=<  OutDataTypeStr=uint8
  Constant : Constant  Value=BatType
  Data Type Conversion1 : DataTypeConversion
  Divide : Product  Inputs=**
  Gain1 : Gain  Gain=Batt.B/3600
  Gain4 : Gain  Gain=Batt.A
  Integrator2 : Integrator  InitialCondition=Batt.A*exp(-Batt.B*(1-SOC/100)*Batt.Q)
  Li-Ion : Fcn  Expr=Batt.A*exp(-Batt.B*u(1))
  Multiport Switch1 : MultiPortSwitch  Inputs=4
  Saturation : Saturate  UpperLimit=Batt.Qmax*(1/Batt.lambda)  LowerLimit=-inf
  Exp : Outport
  wires:
  Integrator2/1 -> Multiport Switch1/2, Multiport Switch1/4, Add3/2, Multiport Switch1/5
  Gain4/1 -> Add3/1
  Divide/1 -> Gain1/1
  Abs/1 -> Divide/1
  Add3/1 -> Divide/2
  Gain1/1 -> Integrator2/1
  i/1 -> Abs/1, Compare To Zero2/1
  Constant/1 -> Multiport Switch1/1
  it/1 -> Saturation/1
  Li-Ion/1 -> Multiport Switch1/3
  Multiport Switch1/1 -> Exp/1
  Compare To Zero2/1 -> Data Type Conversion1/1
  Data Type Conversion1/1 -> Gain4/1
  Saturation/1 -> Li-Ion/1

== system DC_grid_V2/Battery/Model/Power loss estimation ==
  El : Inport
  i : Inport  Port=2
  Memory : Memory
  Product : Product
  Terminator : Terminator
  wires:
  Memory/1 -> Terminator/1
  El/1 -> Product/2
  i/1 -> Product/1
  Product/1 -> Memory/1
